simulink model "TP4"  (R2020a)
settings: Solver=VariableStepAuto  StartTime=0.0  StopTime=20  RelTol=1e-3
values from neighbouring files (symbols this model uses):
  Ki = 64    [TP4_m.m]
  kic = (T.Jeq*omega_n*factores_amortiguamiento)/(T.Nv*(-Sensibilidad_Pitch))    [TP4_m.m]
  Kp = 2.8e-6    (= 2.8e-06)    [TP4_m.m]
  kpc = (2*factores_amortiguamiento*T.Jeq*omega_n)/(T.Nv*(-Sensibilidad_Pitch))    [TP4_m.m]
undefined symbols (not defined in the file or in its folder): G, magnitude, T
libraries: simulink x1
settings Model: Creator=ander  LastModifiedBy=delfi
settings DebuggingCC: SFMachineParentedDataDiag=error  ArithmeticOperatorsInVariantConditions=warning
settings SFSimCC: CustomCodeUndefinedFunction=UseInterfaceOnly
settings CodeAppCC: StateflowObjectComments=on

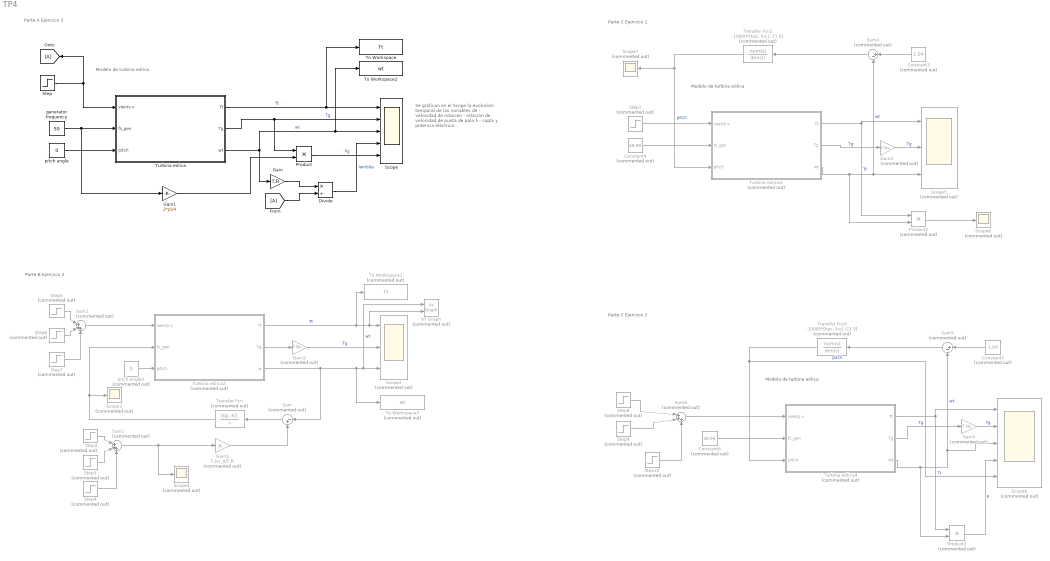
== system TP4 ==
  note: Parte B Ejercicio 2
  note: Se grafican
      | en el Scope la
      | evolución temporal de las
      | variables de
      | - velocidad de rotación
      | - relación de velocidad
      | de punta de pala λ
      | - cupla y potencia eléctrica
  note: Parte A Ejercicio 3
  note: Modelo de turbina eólica
  note: Parte C Ejercicio 1
  note: Modelo de turbina eólica
  note: Parte C Ejercicio 2
  note: Modelo de turbina eólica
  Constant3 : Constant  Commented=on  Value=1.04
  Constant4 : Constant  Commented=on  Value=48.99
  Constant5 : Constant  Commented=on  Value=1.04
  Constant6 : Constant  Commented=on  Value=48.99
  Divide : Product  Inputs=*/
  Gain : Gain  Gain=T.R
  Gain1 : Gain  Gain=2*pi/4
  Gain2 : Gain  Commented=on  Gain=T.Nv
  Gain3 : Gain  Commented=on  Gain=T.tsr_0/T.R
  Gain4 : Gain  Commented=on  Gain=T.Nv
  Gain5 : Gain  Commented=on  Gain=T.Nv
  Product : Product
  Product2 : Product  Commented=on
  Product3 : Product  Commented=on
  Scope : Scope  NumInputPorts=5
  Scope2 : Scope  Commented=on  NumInputPorts=3
  Scope{3..4,6..7} (4 alike) : Scope  Commented=on
  Scope5 : Scope  Commented=on  NumInputPorts=3
  Scope8 : Scope  Commented=on  NumInputPorts=5
  Step : Step  Time=10  Before=5  After=15  SampleTime=0
  Step1 : Step  Commented=on  Time=500  Before=17  After=18  SampleTime=0
  Step10 : Step  Commented=on  Time=750  After=3  SampleTime=0
  Step2 : Step  Commented=on  Time=15  Before=6  After=7  SampleTime=0
  Step3 : Step  Commented=on  Time=30  SampleTime=0
  Step4 : Step  Commented=on  Time=40  After=2  SampleTime=0
  Step5 : Step  Commented=on  Time=15  Before=6  After=7  SampleTime=0
  Step6 : Step  Commented=on  Time=30  SampleTime=0
  Step7 : Step  Commented=on  Time=40  After=2  SampleTime=0
  Step8 : Step  Commented=on  Time=250  Before=13  After=15  SampleTime=0
  Step9 : Step  Commented=on  Time=500  After=3  SampleTime=0
  Sum : Sum  Commented=on  Inputs=|-+
  Sum1 : Sum  Commented=on  Inputs=|+++
  Sum2 : Sum  Commented=on  Inputs=|+++
  Sum4 : Sum  Commented=on  Inputs=|+-
  Sum5 : Sum  Commented=on  Inputs=|+-
  Sum6 : Sum  Commented=on  Inputs=|+++
  To Workspace : ToWorkspace  VariableName=Tt  SampleTime=-1
      settings: Save2DSignal=2-D array (concatenate along first dimension)
  To Workspace1 : ToWorkspace  Commented=on  VariableName=Tt  SampleTime=-1
  To Workspace2 : ToWorkspace  VariableName=wt  SampleTime=-1
      settings: Save2DSignal=2-D array (concatenate along first dimension)
  To Workspace3 : ToWorkspace  Commented=on  VariableName=wt  SampleTime=-1
  Transfer Fcn : TransferFcn  Commented=on  Numerator=[Kp, Ki]  Denominator=[1 0]
  Transfer Fcn2 : TransferFcn  Commented=on  Numerator=-10000*[kpc, kic]  Denominator=[1 0]
  Transfer Fcn3 : TransferFcn  Commented=on  Numerator=-10000*[kpc, kic]  Denominator=[1 0]
  Turbina eólica : Subsystem
  Turbina eólica2 : Subsystem  Commented=on
  Turbina eólica3 : Subsystem  Commented=on
  Turbina eólica4 : Subsystem  Commented=on
  XY Graph : simulink/Sinks/XY Graph  Commented=on  xmin=0  xmax=2  ymin=0  ymax=5e6  st=1
  generator frequency : Constant  Value=50
  pitch angle : Constant  Value=0
  pitch angle2 : Constant  Commented=on  Value=0
  wires:
  Turbina eólica/1(Tt) -> To Workspace/1, Scope/1  "Tt"
  Turbina eólica/2(Tg) -> Product/1, Scope/2  "Tg"
  Turbina eólica/3(wt) -> To Workspace2/1, Scope/3, Gain/1  "wt"
  generator frequency/1 -> Turbina eólica/2(fs_gen), Gain1/1
  pitch angle/1 -> Turbina eólica/3(pitch)
  Step/1 -> Turbina eólica/1(viento v), [A]
  Gain/1 -> Divide/1
  [A] -> Divide/2
  Divide/1 -> Scope/4  "lambda"
  Product/1 -> Scope/5  "Pg"
  Gain1/1 -> Product/2
  Transfer Fcn/1 -> Scope3/1, Turbina eólica2/2(fs_gen)
  Sum1/1 -> Scope4/1, Gain3/1
  Step5/1 -> Sum2/1
  Step4/1 -> Sum1/3
  Turbina eólica2/1(Tt) -> To Workspace1/1, XY Graph/2, Scope2/1  "Tt"
  Sum2/1 -> Turbina eólica2/1(viento v)
  Step7/1 -> Sum2/3
  Step6/1 -> Sum2/2
  Turbina eólica2/2(Tg) -> Gain2/1
  Gain3/1 -> Sum/2
  Step3/1 -> Sum1/2
  Step2/1 -> Sum1/1
  pitch angle2/1 -> Turbina eólica2/3(pitch)
  Gain2/1 -> Scope2/2  "Tg"
  Sum/1 -> Transfer Fcn/1
  Turbina eólica2/3(w) -> Sum/1, To Workspace3/1, XY Graph/1, Scope2/3  "wt"
  Step10/1 -> Sum6/3
  Sum6/1 -> Turbina eólica4/1(viento v)
  Turbina eólica4/1(Tt) -> Product3/1, Scope8/1  "Tt"
  Gain5/1 -> Scope8/2  "Tg"
  Step9/1 -> Sum6/2
  Step8/1 -> Sum6/1
  Constant6/1 -> Turbina eólica4/2(fs_gen)
  Product2/1 -> Scope6/1
  Constant5/1 -> Sum5/1
  Product3/1 -> Scope8/4  "P"
  Transfer Fcn3/1 -> Turbina eólica4/3(pitch), Scope8/5  "pitch"
  Turbina eólica4/3(wt) -> Sum5/2, Scope8/3, Product3/2  "wt"
  Turbina eólica3/1(Tt) -> Product2/1, Scope5/1  "Tt"
  Constant4/1 -> Turbina eólica3/2(fs_gen)
  Sum5/1 -> Transfer Fcn3/1
  Gain4/1 -> Scope5/2  "Tg"
  Step1/1 -> Turbina eólica3/1(viento v)
  Turbina eólica4/2(Tg) -> Gain5/1  "Tg"
  Transfer Fcn2/1 -> Scope7/1, Turbina eólica3/3(pitch)  "pitch"
  Turbina eólica3/3(wt) -> Product2/2, Sum4/2, Scope5/3  "wt"
  Constant3/1 -> Sum4/1
  Turbina eólica3/2(Tg) -> Gain4/1  "Tg"
  Sum4/1 -> Transfer Fcn2/1

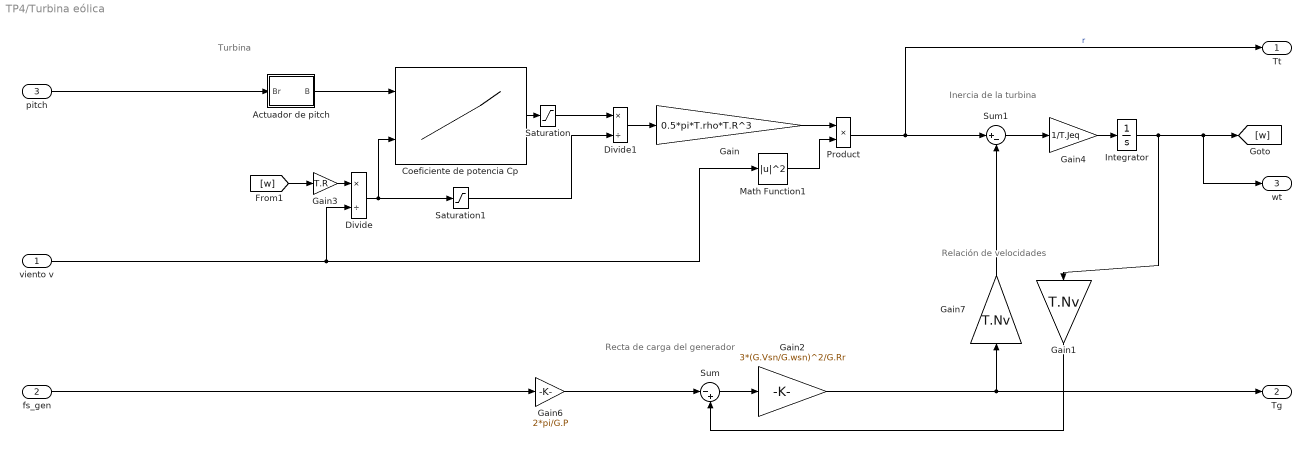
== system TP4/Turbina eólica ==
  note: Relación de velocidades
  note: Turbina
  note: Inercia de la turbina
  note: Recta de carga del generador
  viento v : Inport
  fs_gen : Inport  Port=2
  pitch : Inport  Port=3
  Actuador de pitch : Subsystem
  Coeficiente de potencia Cp : Lookup_n-D  BreakpointsForDimension1=T.pitch  BreakpointsForDimension2=T.tsr  Table=T.Cp  InterpMethod=Cubic spline  InternalRulePriority=Speed  OutMin=[0]  OutMax=[0.5]  RndMeth=Simplest  SaturateOnIntegerOverflow=on  InputSameDT=on
  Divide : Product  Inputs=*/
  Divide1 : Product  Inputs=*/
  Gain : Gain  Gain=0.5*pi*T.rho*T.R^3
  Gain1 : Gain  Gain=T.Nv
  Gain2 : Gain  Gain=3*(G.Vsn/G.wsn)^2/G.Rr
  Gain3 : Gain  Gain=T.R
  Gain4 : Gain  Gain=1/T.Jeq
  Gain6 : Gain  Gain=2*pi/G.P
  Gain7 : Gain  Gain=T.Nv
  Integrator : Integrator  InitialCondition=G.wsn/T.Nv
  Math Function1 : Math  Operator=magnitude^2  SignedPower=on  SaturateOnIntegerOverflow=on
  Product : Product
  Saturation : Saturate  LowerLimit=0
  Saturation1 : Saturate  UpperLimit=inf  LowerLimit=0.1
  Sum : Sum  Inputs=|-+
  Sum1 : Sum  Inputs=|+-
  Tt : Outport
  Tg : Outport  Port=2
  wt : Outport  Port=3
  wires:
  Coeficiente de potencia Cp/1 -> Saturation/1
  fs_gen/1 -> Gain6/1
  Divide/1 -> Coeficiente de potencia Cp/2, Saturation1/1
  Integrator/1 -> Gain1/1, wt/1, [w]
  Gain3/1 -> Divide/1
  viento v/1 -> Divide/2, Math Function1/1
  Product/1 -> Tt/1, Sum1/1  "r"
  Gain2/1 -> Tg/1, Gain7/1
  Sum1/1 -> Gain4/1
  Gain7/1 -> Sum1/2
  [w] -> Gain3/1
  Math Function1/1 -> Product/2
  Saturation1/1 -> Divide1/2
  Saturation/1 -> Divide1/1
  Gain1/1 -> Sum/2
  Sum/1 -> Gain2/1
  Divide1/1 -> Gain/1
  Gain/1 -> Product/1
  Gain4/1 -> Integrator/1
  Gain6/1 -> Sum/1
  pitch/1 -> Actuador de pitch/1(Br)
  Actuador de pitch/1(B) -> Coeficiente de potencia Cp/1

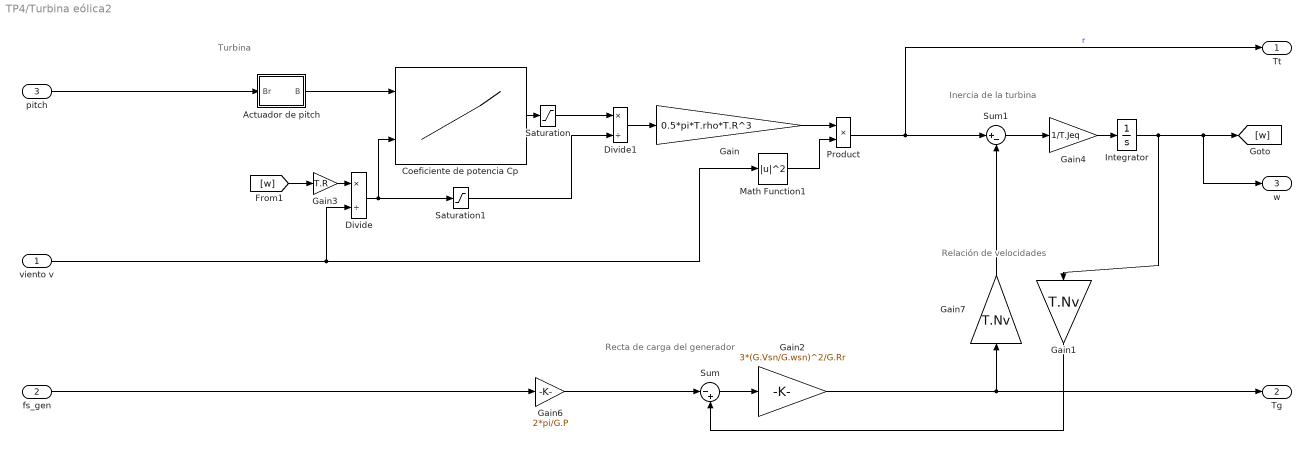
== system TP4/Turbina eólica2 ==
  note: Relación de velocidades
  note: Turbina
  note: Inercia de la turbina
  note: Recta de carga del generador
  viento v : Inport
  fs_gen : Inport  Port=2
  pitch : Inport  Port=3
  Actuador de pitch : Subsystem
  Coeficiente de potencia Cp : Lookup_n-D  BreakpointsForDimension1=T.pitch  BreakpointsForDimension2=T.tsr  Table=T.Cp  InterpMethod=Cubic spline  InternalRulePriority=Speed  OutMin=[0]  OutMax=[0.5]  RndMeth=Simplest  SaturateOnIntegerOverflow=on  InputSameDT=on
  Divide : Product  Inputs=*/
  Divide1 : Product  Inputs=*/
  Gain : Gain  Gain=0.5*pi*T.rho*T.R^3
  Gain1 : Gain  Gain=T.Nv
  Gain2 : Gain  Gain=3*(G.Vsn/G.wsn)^2/G.Rr
  Gain3 : Gain  Gain=T.R
  Gain4 : Gain  Gain=1/T.Jeq
  Gain6 : Gain  Gain=2*pi/G.P
  Gain7 : Gain  Gain=T.Nv
  Integrator : Integrator  InitialCondition=G.wsn/T.Nv
  Math Function1 : Math  Operator=magnitude^2  SignedPower=on  SaturateOnIntegerOverflow=on
  Product : Product
  Saturation : Saturate  LowerLimit=0
  Saturation1 : Saturate  UpperLimit=inf  LowerLimit=0.1
  Sum : Sum  Inputs=|-+
  Sum1 : Sum  Inputs=|+-
  Tt : Outport
  Tg : Outport  Port=2
  w : Outport  Port=3
  wires:
  Coeficiente de potencia Cp/1 -> Saturation/1
  fs_gen/1 -> Gain6/1
  Divide/1 -> Coeficiente de potencia Cp/2, Saturation1/1
  Integrator/1 -> Gain1/1, w/1, [w]
  Gain3/1 -> Divide/1
  viento v/1 -> Divide/2, Math Function1/1
  Product/1 -> Tt/1, Sum1/1  "r"
  Gain2/1 -> Tg/1, Gain7/1
  Sum1/1 -> Gain4/1
  Gain7/1 -> Sum1/2
  [w] -> Gain3/1
  Math Function1/1 -> Product/2
  Saturation1/1 -> Divide1/2
  pitch/1 -> Actuador de pitch/1(Br)
  Saturation/1 -> Divide1/1
  Gain1/1 -> Sum/2
  Sum/1 -> Gain2/1
  Actuador de pitch/1(B) -> Coeficiente de potencia Cp/1
  Divide1/1 -> Gain/1
  Gain/1 -> Product/1
  Gain4/1 -> Integrator/1
  Gain6/1 -> Sum/1

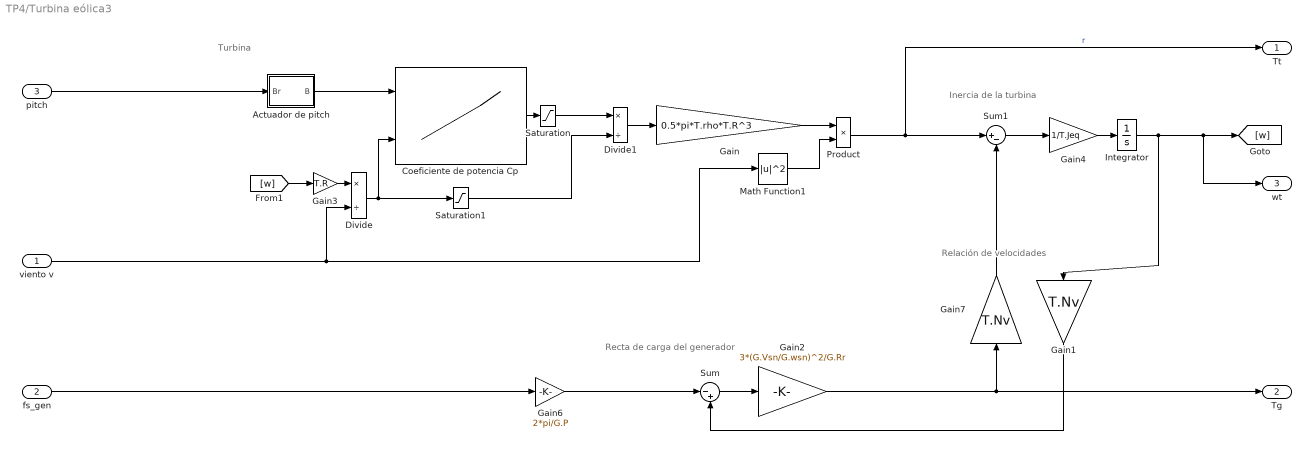
== system TP4/Turbina eólica3 ==
  note: Relación de velocidades
  note: Turbina
  note: Inercia de la turbina
  note: Recta de carga del generador
  viento v : Inport
  fs_gen : Inport  Port=2
  pitch : Inport  Port=3
  Actuador de pitch : Subsystem
  Coeficiente de potencia Cp : Lookup_n-D  BreakpointsForDimension1=T.pitch  BreakpointsForDimension2=T.tsr  Table=T.Cp  InterpMethod=Cubic spline  InternalRulePriority=Speed  OutMin=[0]  OutMax=[0.5]  RndMeth=Simplest  SaturateOnIntegerOverflow=on  InputSameDT=on
  Divide : Product  Inputs=*/
  Divide1 : Product  Inputs=*/
  Gain : Gain  Gain=0.5*pi*T.rho*T.R^3
  Gain1 : Gain  Gain=T.Nv
  Gain2 : Gain  Gain=3*(G.Vsn/G.wsn)^2/G.Rr
  Gain3 : Gain  Gain=T.R
  Gain4 : Gain  Gain=1/T.Jeq
  Gain6 : Gain  Gain=2*pi/G.P
  Gain7 : Gain  Gain=T.Nv
  Integrator : Integrator  InitialCondition=G.wsn/T.Nv
  Math Function1 : Math  Operator=magnitude^2  SignedPower=on  SaturateOnIntegerOverflow=on
  Product : Product
  Saturation : Saturate  LowerLimit=0
  Saturation1 : Saturate  UpperLimit=inf  LowerLimit=0.1
  Sum : Sum  Inputs=|-+
  Sum1 : Sum  Inputs=|+-
  Tt : Outport
  Tg : Outport  Port=2
  wt : Outport  Port=3
  wires:
  Coeficiente de potencia Cp/1 -> Saturation/1
  fs_gen/1 -> Gain6/1
  Divide/1 -> Coeficiente de potencia Cp/2, Saturation1/1
  Integrator/1 -> Gain1/1, wt/1, [w]
  Gain3/1 -> Divide/1
  viento v/1 -> Divide/2, Math Function1/1
  Product/1 -> Tt/1, Sum1/1  "r"
  Gain2/1 -> Tg/1, Gain7/1
  Sum1/1 -> Gain4/1
  Gain7/1 -> Sum1/2
  [w] -> Gain3/1
  Math Function1/1 -> Product/2
  Saturation1/1 -> Divide1/2
  Saturation/1 -> Divide1/1
  Gain1/1 -> Sum/2
  Sum/1 -> Gain2/1
  Divide1/1 -> Gain/1
  Gain/1 -> Product/1
  Gain4/1 -> Integrator/1
  Gain6/1 -> Sum/1
  pitch/1 -> Actuador de pitch/1(Br)
  Actuador de pitch/1(B) -> Coeficiente de potencia Cp/1

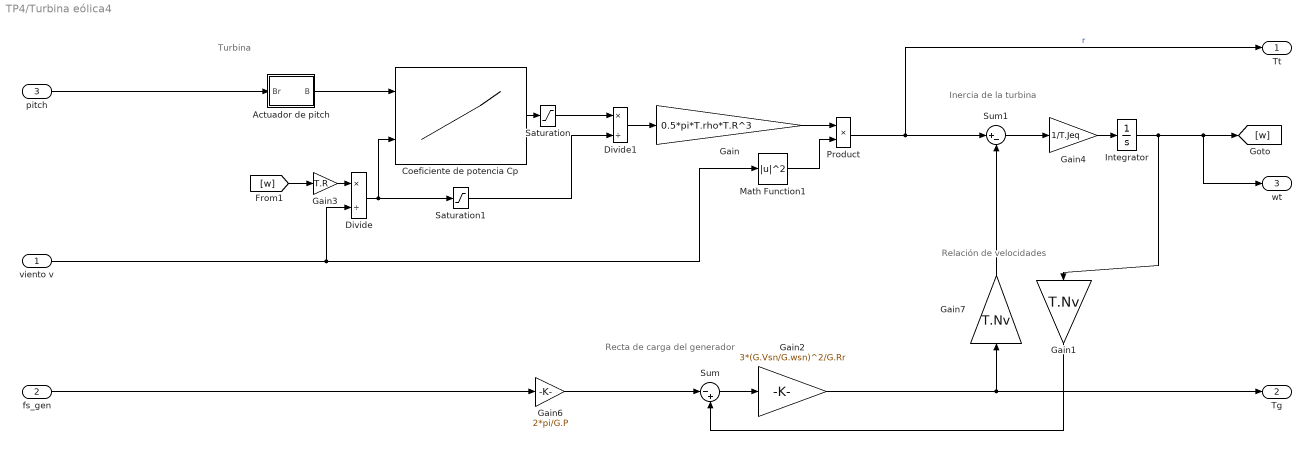
== system TP4/Turbina eólica4 ==
  note: Relación de velocidades
  note: Turbina
  note: Inercia de la turbina
  note: Recta de carga del generador
  viento v : Inport
  fs_gen : Inport  Port=2
  pitch : Inport  Port=3
  Actuador de pitch : Subsystem
  Coeficiente de potencia Cp : Lookup_n-D  BreakpointsForDimension1=T.pitch  BreakpointsForDimension2=T.tsr  Table=T.Cp  InterpMethod=Cubic spline  InternalRulePriority=Speed  OutMin=[0]  OutMax=[0.5]  RndMeth=Simplest  SaturateOnIntegerOverflow=on  InputSameDT=on
  Divide : Product  Inputs=*/
  Divide1 : Product  Inputs=*/
  Gain : Gain  Gain=0.5*pi*T.rho*T.R^3
  Gain1 : Gain  Gain=T.Nv
  Gain2 : Gain  Gain=3*(G.Vsn/G.wsn)^2/G.Rr
  Gain3 : Gain  Gain=T.R
  Gain4 : Gain  Gain=1/T.Jeq
  Gain6 : Gain  Gain=2*pi/G.P
  Gain7 : Gain  Gain=T.Nv
  Integrator : Integrator  InitialCondition=G.wsn/T.Nv
  Math Function1 : Math  Operator=magnitude^2  SignedPower=on  SaturateOnIntegerOverflow=on
  Product : Product
  Saturation : Saturate  LowerLimit=0
  Saturation1 : Saturate  UpperLimit=inf  LowerLimit=0.1
  Sum : Sum  Inputs=|-+
  Sum1 : Sum  Inputs=|+-
  Tt : Outport
  Tg : Outport  Port=2
  wt : Outport  Port=3
  wires:
  Coeficiente de potencia Cp/1 -> Saturation/1
  fs_gen/1 -> Gain6/1
  Divide/1 -> Coeficiente de potencia Cp/2, Saturation1/1
  Integrator/1 -> Gain1/1, wt/1, [w]
  Gain3/1 -> Divide/1
  viento v/1 -> Divide/2, Math Function1/1
  Product/1 -> Tt/1, Sum1/1  "r"
  Gain2/1 -> Tg/1, Gain7/1
  Sum1/1 -> Gain4/1
  Gain7/1 -> Sum1/2
  [w] -> Gain3/1
  Math Function1/1 -> Product/2
  Saturation1/1 -> Divide1/2
  Saturation/1 -> Divide1/1
  Gain1/1 -> Sum/2
  Sum/1 -> Gain2/1
  Divide1/1 -> Gain/1
  Gain/1 -> Product/1
  Gain4/1 -> Integrator/1
  Gain6/1 -> Sum/1
  pitch/1 -> Actuador de pitch/1(Br)
  Actuador de pitch/1(B) -> Coeficiente de potencia Cp/1

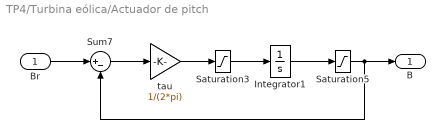
== system TP4/Turbina eólica/Actuador de pitch ==
  Br : Inport
  Integrator1 : Integrator
  Saturation3 : Saturate  UpperLimit=10  LowerLimit=-10
  Saturation5 : Saturate  UpperLimit=30  LowerLimit=0
  Sum7 : Sum  Inputs=|+-
  tau : Gain  Gain=1/(2*pi)
  B : Outport
  wires:
  Saturation5/1 -> B/1, Sum7/2
  Integrator1/1 -> Saturation5/1
  tau/1 -> Saturation3/1
  Saturation3/1 -> Integrator1/1
  Sum7/1 -> tau/1
  Br/1 -> Sum7/1

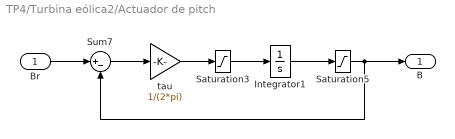
== system TP4/Turbina eólica2/Actuador de pitch ==
  Br : Inport
  Integrator1 : Integrator
  Saturation3 : Saturate  UpperLimit=10  LowerLimit=-10
  Saturation5 : Saturate  UpperLimit=30  LowerLimit=0
  Sum7 : Sum  Inputs=|+-
  tau : Gain  Gain=1/(2*pi)
  B : Outport
  wires:
  Saturation5/1 -> B/1, Sum7/2
  Br/1 -> Sum7/1
  Integrator1/1 -> Saturation5/1
  tau/1 -> Saturation3/1
  Saturation3/1 -> Integrator1/1
  Sum7/1 -> tau/1

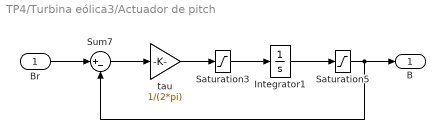
== system TP4/Turbina eólica3/Actuador de pitch ==
  Br : Inport
  Integrator1 : Integrator
  Saturation3 : Saturate  UpperLimit=10  LowerLimit=-10
  Saturation5 : Saturate  UpperLimit=30  LowerLimit=0
  Sum7 : Sum  Inputs=|+-
  tau : Gain  Gain=1/(2*pi)
  B : Outport
  wires:
  Saturation5/1 -> B/1, Sum7/2
  Integrator1/1 -> Saturation5/1
  tau/1 -> Saturation3/1
  Saturation3/1 -> Integrator1/1
  Sum7/1 -> tau/1
  Br/1 -> Sum7/1

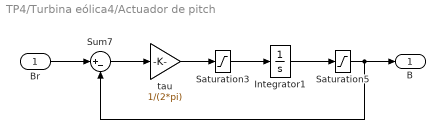
== system TP4/Turbina eólica4/Actuador de pitch ==
  Br : Inport
  Integrator1 : Integrator
  Saturation3 : Saturate  UpperLimit=10  LowerLimit=-10
  Saturation5 : Saturate  UpperLimit=30  LowerLimit=0
  Sum7 : Sum  Inputs=|+-
  tau : Gain  Gain=1/(2*pi)
  B : Outport
  wires:
  Saturation5/1 -> B/1, Sum7/2
  Integrator1/1 -> Saturation5/1
  tau/1 -> Saturation3/1
  Saturation3/1 -> Integrator1/1
  Sum7/1 -> tau/1
  Br/1 -> Sum7/1
